simulink subsystem "h_bridge"  (R2023a)
settings: Solver=VariableStepAuto  StartTime=0.0  StopTime=10.0  RelTol=1e-3
libraries: fl_lib x1, eeGeneralControl x1, nesl_utility x1
settings Model: Creator=motya  LastModifiedBy=motya

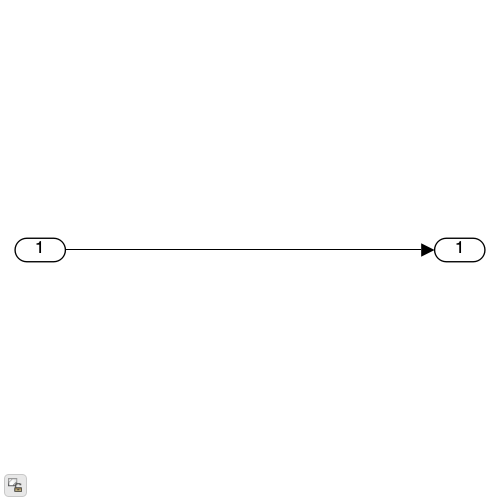
[thumbnail: Simulink's stored preview of the top-level diagram]
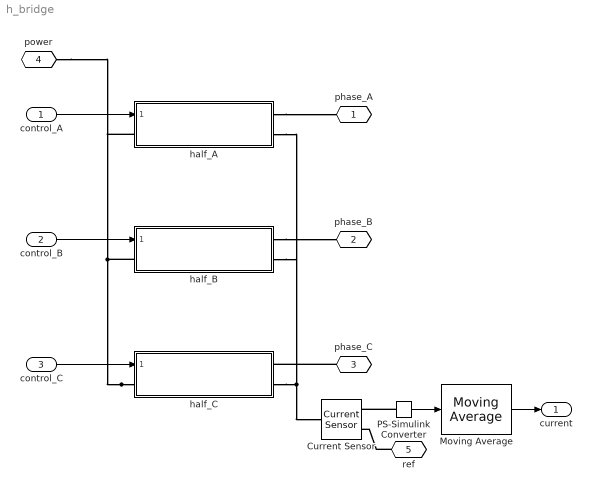
== system h_bridge ==
  control_A : Inport
  control_B : Inport  Port=2
  control_C : Inport  Port=3
  Current Sensor : fl_lib/Electrical/Electrical Sensors/Current Sensor
  Moving Average : eeGeneralControl/Moving Average  VariantControl=Variant1  LabelModeActiveChoice=Discrete  f=60  x0=0  BufferSize=8192  Ts=-1
      settings: LibrarySourceBlock=ee_sl_lib/General Control/Moving Average
  PS-Simulink Converter : nesl_utility/PS-Simulink Converter  PhysicalDomain=network_engine_domain  SubClassName=ps_output  LeftPortType=input  RightPortType=output  PseudoPeriodic=off  Frequencies=[]  VectorFormat=inherit  Unit=inherit  AffineConversion=off
  half_A : Subsystem  ReferencedSubsystem=half_bridge
  half_B : Subsystem  ReferencedSubsystem=half_bridge
  half_C : Subsystem  ReferencedSubsystem=half_bridge
  phase_A : PMIOPort  Side=Right
  phase_B : PMIOPort  Port=2  Side=Right
  phase_C : PMIOPort  Port=3  Side=Right
  power : PMIOPort  Port=4  Side=Left
  ref : PMIOPort  Port=5  Side=Right
  current : Outport
  wires:
  control_A/1 -> half_A/1
  control_B/1 -> half_B/1
  control_C/1 -> half_C/1
  Moving Average/1 -> current/1
  PS-Simulink Converter/1 -> Moving Average/1
  connections:
  half_C/LConn1 -- power/RConn1 -- half_A/LConn1 -- half_B/LConn1
  half_C/RConn2 -- Current Sensor/LConn1 -- half_A/RConn2 -- half_B/RConn2
  half_A/RConn1 -- phase_A/RConn1
  half_B/RConn1 -- phase_B/RConn1
  phase_C/RConn1 -- half_C/RConn1
  PS-Simulink Converter/LConn1 -- Current Sensor/RConn1
  ref/RConn1 -- Current Sensor/RConn2
